simulink model "Ex10_4_1_RocketPropelledSled"  (R2023a)
settings: Solver=VariableStepAuto  StartTime=0.0  StopTime=10.0  RelTol=1e-3
settings Model: Creator=Norb  LastModifiedBy=Norb

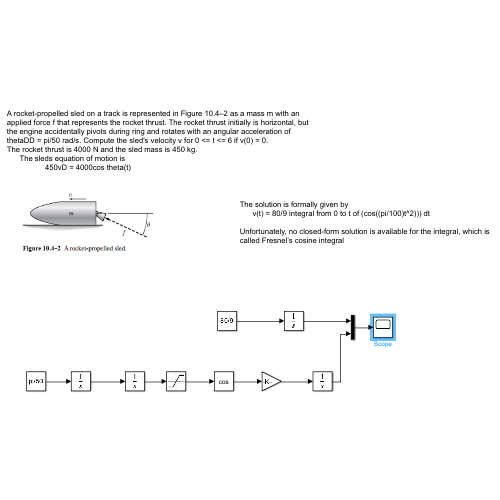
[thumbnail: Simulink's stored preview of the top-level diagram]
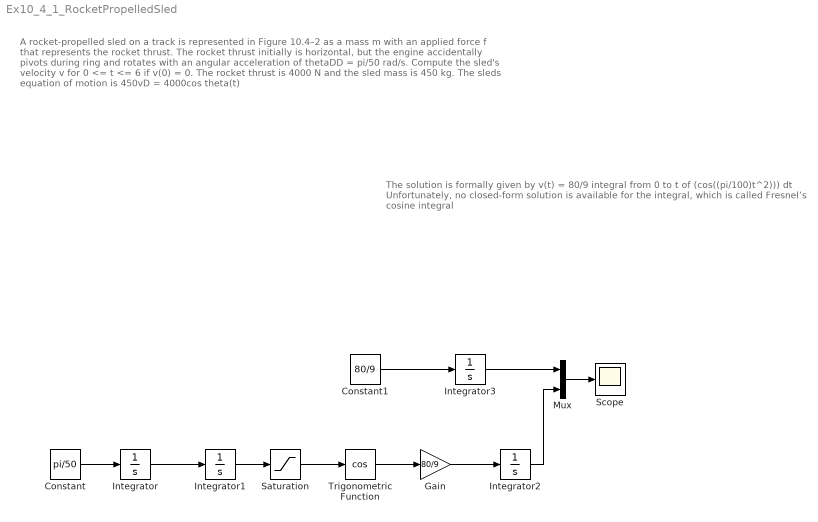
== system Ex10_4_1_RocketPropelledSled ==
  note: The solution is formally given by
      | v(t) = 80/9 integral from 0 to t of (cos((pi/100)t^2))) dt
      |
      | Unfortunately, no closed-form solution is available for the integral, which is called Fresnel’s cosine integral
  note: A rocket-propelled sled on a track is represented in Figure 10.4–2 as a mass m with an applied force f that represents the rocket thrust. The rocket thrust initially is horizontal, but the engine accidentally pivots during ring and rotates with an angular acceleration of
      | thetaDD = pi/50 rad/s. Compute the sled's velocity v for 0 <= t <= 6 if v(0) = 0.
      | The rocket thrust is 4000 N and the sled mass is 450 kg.
      | The sleds equation of motion is
      | 450vD = 4000cos theta(t)
  Constant : Constant  Value=pi/50
  Constant1 : Constant  Value=80/9
  Gain : Gain  Gain=80/9
  Integrator{,1..3} (4 alike) : Integrator
  Mux : Mux  Inputs=2
  Saturation : Saturate  UpperLimit=(60*pi)/180  LowerLimit=0
  Scope : Scope
  Trigonometric Function : Trigonometry  Operator=cos
  wires:
  Constant/1 -> Integrator/1
  Integrator/1 -> Integrator1/1
  Integrator1/1 -> Saturation/1
  Trigonometric Function/1 -> Gain/1
  Gain/1 -> Integrator2/1
  Integrator2/1 -> Mux/2
  Saturation/1 -> Trigonometric Function/1
  Mux/1 -> Scope/1
  Constant1/1 -> Integrator3/1
  Integrator3/1 -> Mux/1
